simulink subsystem "Brayton_ROM"  (R2023a)
settings: Solver=VariableStepAuto  StartTime=0.0  StopTime=10.0  RelTol=1e-3
undefined symbols (not defined in the file): initT3, phiMean, phiStd, powerMean, powerStd, rpm0, RPM_refMean, RPM_refStd, rpmMean, rpmStd, t3Mean, t3Std
libraries: deeplib x1
settings Model: Creator=imyrsini  LastModifiedBy=imyrsini

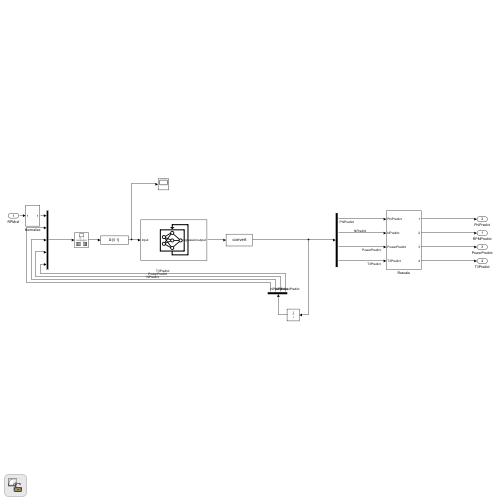
[thumbnail: Simulink's stored preview of the top-level diagram]
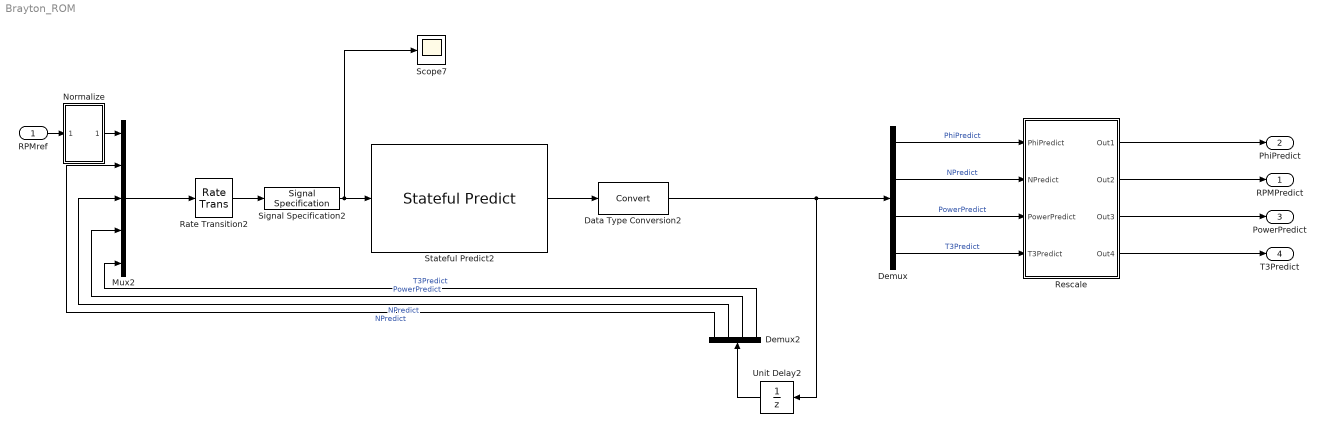
== system Brayton_ROM ==
  RPMref : Inport
  Data Type Conversion2 : DataTypeConversion  SaturateOnIntegerOverflow=off  RndMeth=Floor
  Demux : Demux
  Demux2 : Demux
  Mux2 : Mux  Inputs=5
  Normalize : Subsystem
  Rate Transition2 : RateTransition  OutPortSampleTime=samplTime
  Rescale : Subsystem
  Scope7 : Scope
  Signal Specification2 : SignalSpecification  Dimensions=[5 1]
  Stateful Predict2 : deeplib/Stateful Predict  Network=Network from MAT-file  NetworkFunction=untitled  NetworkFilePath=C:\Users\imyrsini\OneDrive - MathWorks\Documents\Projects\AEprojects\LSTM Model Reduction\BraytonGasTurbSimplified_LSTMReductionTrial\braytonLSTMNetThermoNorm.mat  InputDataFormats={'',''}  SampleTime=-1  ForceInterpretedSim=off  EnableDLNetwork=on
  Unit Delay2 : UnitDelay  InitialCondition=[0; (rpm0-rpmMean)/rpmStd; 0; (initT3-t3Mean)/t3Std]  SampleTime=-1  HasFrameUpgradeWarning=on
  RPMPredict : Outport
  PhiPredict : Outport  Port=2
  PowerPredict : Outport  Port=3
  T3Predict : Outport  Port=4
  wires:
  Demux2/3 -> Mux2/4  "PowerPredict"
  Stateful Predict2/1 -> Data Type Conversion2/1
  Rate Transition2/1 -> Signal Specification2/1
  Demux2/4 -> Mux2/5  "T3Predict"
  Unit Delay2/1 -> Demux2/1
  Demux2/2 -> Mux2/3  "NPredict"
  Signal Specification2/1 -> Scope7/1, Stateful Predict2/1
  Demux2/1 -> Mux2/2  "NPredict"
  Demux/1 -> Rescale/1(PhiPredict)  "PhiPredict"
  Demux/2 -> Rescale/2(NPredict)  "NPredict"
  Demux/3 -> Rescale/3(PowerPredict)  "PowerPredict"
  Demux/4 -> Rescale/4(T3Predict)  "T3Predict"
  Rescale/1(Out1) -> PhiPredict/1
  Rescale/2(Out2) -> RPMPredict/1
  Rescale/3(Out3) -> PowerPredict/1
  Rescale/4(Out4) -> T3Predict/1
  Data Type Conversion2/1 -> Demux/1, Unit Delay2/1
  Mux2/1 -> Rate Transition2/1
  RPMref/1 -> Normalize/1(In1)
  Normalize/1(Out1) -> Mux2/1

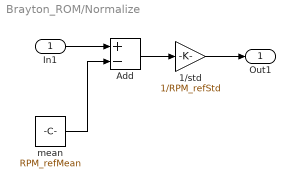
== system Brayton_ROM/Normalize ==
  In1 : Inport
  1/std : Gain  Gain=1/RPM_refStd
  Add : Sum  Inputs=+-
  mean : Constant  Value=RPM_refMean
  Out1 : Outport
  wires:
  1/std/1 -> Out1/1
  mean/1 -> Add/2
  Add/1 -> 1/std/1
  In1/1 -> Add/1

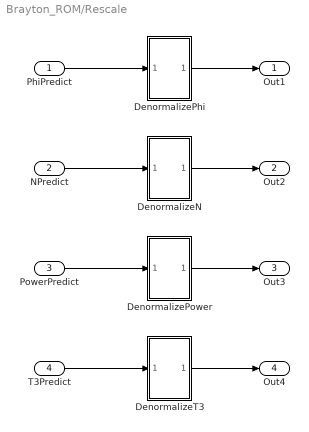
== system Brayton_ROM/Rescale ==
  PhiPredict : Inport
  NPredict : Inport  Port=2
  PowerPredict : Inport  Port=3
  T3Predict : Inport  Port=4
  DenormalizeN : Subsystem
  DenormalizePhi : Subsystem
  DenormalizePower : Subsystem
  DenormalizeT3 : Subsystem
  Out1 : Outport
  Out2 : Outport  Port=2
  Out3 : Outport  Port=3
  Out4 : Outport  Port=4
  wires:
  DenormalizeT3/1(Out1) -> Out4/1
  DenormalizePower/1(Out1) -> Out3/1
  DenormalizeN/1(Out1) -> Out2/1
  DenormalizePhi/1(Out1) -> Out1/1
  PhiPredict/1 -> DenormalizePhi/1(PhiPredict)
  PowerPredict/1 -> DenormalizePower/1(PowerPredict)
  T3Predict/1 -> DenormalizeT3/1(T3Predict)
  NPredict/1 -> DenormalizeN/1(NPredict)

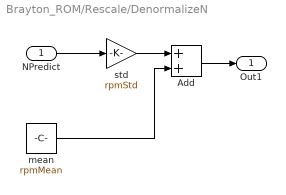
== system Brayton_ROM/Rescale/DenormalizeN ==
  NPredict : Inport
  Add : Sum
  mean : Constant  Value=rpmMean
  std : Gain  Gain=rpmStd
  Out1 : Outport
  wires:
  NPredict/1 -> std/1
  mean/1 -> Add/2
  std/1 -> Add/1
  Add/1 -> Out1/1

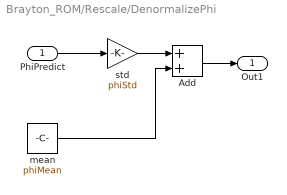
== system Brayton_ROM/Rescale/DenormalizePhi ==
  PhiPredict : Inport
  Add : Sum
  mean : Constant  Value=phiMean
  std : Gain  Gain=phiStd
  Out1 : Outport
  wires:
  Add/1 -> Out1/1
  std/1 -> Add/1
  mean/1 -> Add/2
  PhiPredict/1 -> std/1

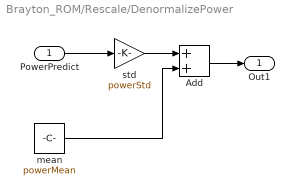
== system Brayton_ROM/Rescale/DenormalizePower ==
  PowerPredict : Inport
  Add : Sum
  mean : Constant  Value=powerMean
  std : Gain  Gain=powerStd
  Out1 : Outport
  wires:
  Add/1 -> Out1/1
  std/1 -> Add/1
  mean/1 -> Add/2
  PowerPredict/1 -> std/1

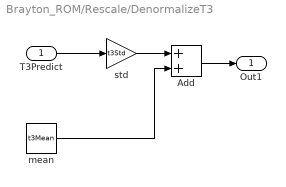
== system Brayton_ROM/Rescale/DenormalizeT3 ==
  T3Predict : Inport
  Add : Sum
  mean : Constant  Value=t3Mean
  std : Gain  Gain=t3Std
  Out1 : Outport
  wires:
  T3Predict/1 -> std/1
  mean/1 -> Add/2
  std/1 -> Add/1
  Add/1 -> Out1/1
